simulink model "SimulinkRobot_Test0_FwdDyn"  (R2023b)
settings: Solver=VariableStepAuto  StartTime=0.0  StopTime=5  RelTol=1e-3
values from neighbouring files (symbols this model uses):
  grav = [0;0;0;0;0;-9.8]    [regressorTest.m]
undefined symbols (not defined in the file or in its folder): Mlist, TfLists, Twists
settings Model: Creator=mechmedic  LastModifiedBy=mechmedic

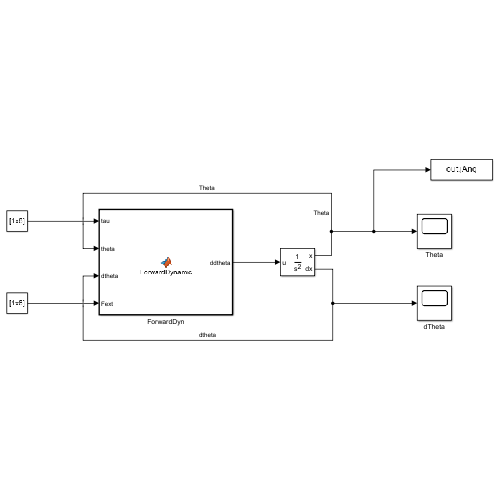
[thumbnail: Simulink's stored preview of the top-level diagram]
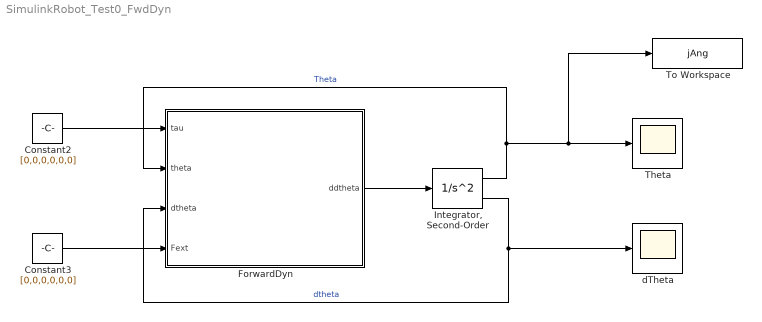
== system SimulinkRobot_Test0_FwdDyn ==
  Constant2 : Constant  Value=[0,0,0,0,0,0]
  Constant3 : Constant  Value=[0,0,0,0,0,0]
  ForwardDyn : MATLAB Function  TreatAsAtomicUnit=on
  "Integrator, Second-Order" : SecondOrderIntegrator
  Theta : Scope
  To Workspace : ToWorkspace  VariableName=jAng  SaveFormat=Timeseries  SampleTime=-1
  dTheta : Scope
  wires:
  Constant3/1 -> ForwardDyn/4(Fext)
  ForwardDyn/1(ddtheta) -> "Integrator, Second-Order"/1
  "Integrator, Second-Order"/1 -> ForwardDyn/2(theta), To Workspace/1, Theta/1  "Theta"
  "Integrator, Second-Order"/2 -> dTheta/1, ForwardDyn/3(dtheta)  "dtheta"
  Constant2/1 -> ForwardDyn/1(tau)

== matlab function SimulinkRobot_Test0_FwdDyn/ForwardDyn ==
  settings: sampleTime=0.01
  data: tau input size=[6 1]; theta input double size=[6 1]; dtheta input double size=[6 1]; Fext input; Twists parameter size=size(Twists); TfLists parameter size=size(TfLists); ddtheta output double size=[6 1]; Mlist parameter size=size(Mlist); grav parameter size=size(grav)
function ddtheta =  ForwardDynamic (tau, theta, dtheta, Fext, Twists, TfLists, Mlist, grav)
    ddtheta =  FwdDyn(tau, theta, dtheta, Fext, Twists, TfLists, Mlist, grav);
